simulink model "MJAUV_Maneuverability_model_V2"  (R2022b)
settings: Solver=ode4  StartTime=0.0  StopTime=50  FixedStep=0.0001  RelTol=1e-3  EnableMultiTasking=on
libraries: sharedutil x64, matrix_library x35
(part 1 of 5)
settings Model: Creator=Waqas Ali Waqar  LastModifiedBy=Administrator
settings SolverCC: ConcurrentTasks=on  ZeroCrossAlgorithm=Adaptive  AutoInsertRateTranBlk=on  InsertRTBMode=Never (minimum delay)
settings DataIOCC: SaveFormat=StructureWithTime
settings OptimizationCC: BlockReduction=off  OptimizeBlockIOStorage=off  BufferReuse=off  GlobalBufferReuse=off  ExpressionFolding=off  PassReuseOutputArgsThreshold=0  LocalBlockOutputs=off  OptimizeBlockOrder=speed  OptimizeDataStoreBuffers=off  BusAssignmentInplaceUpdate=off
settings DebuggingCC: IgnoredZcDiagnostic=none  ParameterTunabilityLossMsg=error  UnconnectedInputMsg=warning  UnconnectedOutputMsg=warning  UnconnectedLineMsg=warning
settings HardwareCC: ProdBitPerPointer=32  ProdBitPerSizeT=32  ProdBitPerPtrDiffT=32  ProdLargestAtomicFloat=None  ProdWordSize=32  ProdLongLongMode=on  ProdHWDeviceType=Generic->32-bit x86 compatible
settings ModelReferenceCC: EnableRefExpFcnMdlSchedulingChecks=on
settings SFSimCC: MATLABDynamicMemAlloc=off  CustomCodeUndefinedFunction=UseInterfaceOnly
settings RTWCC: GenerateReport=on  RTWVerbose=off  LaunchReport=on  RTWCompilerOptimization=on  DLArmComputeVersion=19.05
settings CodeAppCC: ForceParamTrailComments=on  OperatorAnnotations=on
settings GRTTargetCC: TargetLangStandard=C89/C90 (ANSI)

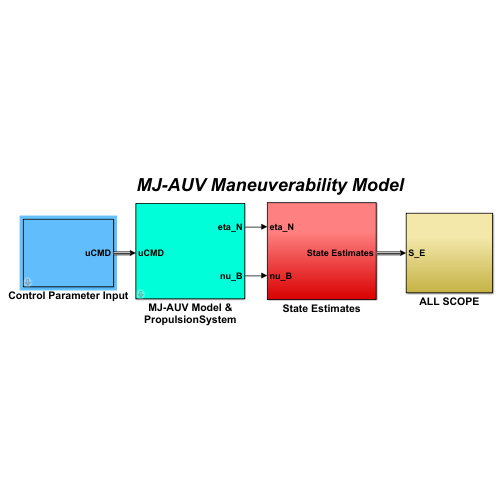
[thumbnail: Simulink's stored preview of the top-level diagram]
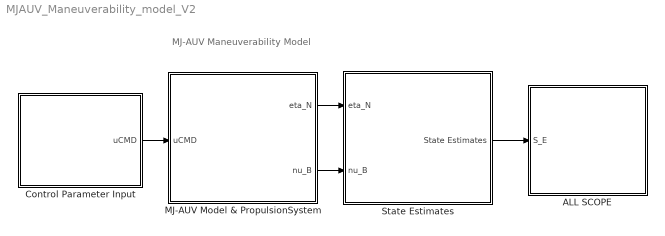
== system MJAUV_Maneuverability_model_V2 ==
  note: MJ-AUV Maneuverability Model
  ALL SCOPE : Subsystem
  Control Parameter Input : Subsystem  mask{uHT=50, uVT1=0, uVT2=0, Theta1=pi/60, Theta2=pi/60, Theta3=pi/60, x_rG_S=0, y_rG_S=0, z_rG_S=0, Delta_B_T=-2}
      mask prompts: uHT "uHT (rps)"; uVT1 "uVT1 (rad)"; uVT2 "uVT2 (rad)"; Theta1 "Theta1 (rad)"; Theta2 "Theta2 (rad)"; Theta3 "Theta3 (rad)"; Delta_B_T "Delta_B_T (N)"
      mask DialogControl ParameterGroupVar Prompt: Control Parameter Input
      mask DialogControl Container3 Prompt: rG_S
  MJ-AUV Model & PropulsionSystem : Subsystem  mask{R=0.15, rho=1025, g=9.8, cdf=0.5, cdt=1, DL=diag([0;0;0;0;0;0]), e1=[1;0;0], e2=[0;1;0], e3=[0;0;1], mB=38.58, IB=[0.434 0 0;0 1.126 0;0 0 1.126], LB=0.532, rG_B=[0;0;0], rB_B=[0;0;-0.01], l_B=[-0.532;0;0], r_B=[-0.532/2;0;0], B_B=377.7, W_B=377.7, mS=50.862, IS=[0.572 0 0;0 2.375 0;0 0 2.375], LS=0.702, rB_S=[0;0;-0.01], l_S=[-0.702;0;0], r_S=[-0.702/2;0;0], B_S=498.45, W_S=498.45, mT=50.862, IT=[0.572 0 0;0 2.375 0;0 0 2.375], LT=0.702, rG_T=[0;0;0], rB_T=[0;0;-0.01], l_T=[-0.702;0;0], r_T=[-0.702/2;0;0], W_T=498.45, mF=23.185, IF=[0.261 0 0;0 1.067 0;0 0 1.067], LF=0.320, rG_F=[0;0;0], rB_F=[0;0;-0.01], l_F=[-0.320;0;0], r_F=[-0.320/2;0;0], B_F=227.213, W_F=227.213, cL=0.5, xfin=-0.03, yfin=0.325, zfin=-0.045, alpha=0, Sfin=0.0421, r1=[-0.16;0;0], D=0.0762}
      mask prompts: R "Body Radius R"; rho "Seawater Density rho"; g "Acceleration of Gravity g"; cdf "Axial Drag Coefficient cdf"; cdt "Radial Drag Coefficient  cdt [0.8-1.2]"; DL "Linear Damping Matrix"; mB "Mass mB"; IB "Inertia Tensor IB"; LB "Length LB"; B_B "Buoyancy"; W_B "Weight"; mS "Mass mS"; IS "Inertia Tensor IS"; LS "Length LS"; rB_S "rB_B"; B_S "Buoyancy"; W_S "Weight"; mT "Mass mT"; IT "Inertia Tensor IT"; LT "Length LT"; W_T "Weight"; mF "Mass mF"; IF "Inertia Tensor IF"; LF "Length LF"; B_F "Buoyancy"; W_F "Weight"; cL "fin lift coefficient  cL:"; xfin "fin axial position xfin:"; yfin "fin axial position yfin:"; zfin "fin axial position zfin:"; alpha "fin flutter angle alpha"; Sfin "fin platform area Sfin:"; D "Diameter"
      mask init:
      | %%%%%%%%%%%%%%%%%%%%%%%%%%%%%%%%%%%%%%%%%%%%%%%%%%%%%%%
      | %%%%%%%%%%%%%%%%%%%  动力学  %%%%%%%%%%%%%%%%%%%%%%%%
      | %%%%%%%%%%%%%%%%%%%%%%%%%%%%%%%%%%%%%%%%%%%%%%%%%%%%%%%
      | 
      | 
      | %% JOINT-1
      | % 粘性水动力系数
      | Af = pi*R^2;
      | At_B = 2*pi*R*LB;
      | 
      | X_uu_B = rho*Af*cdf/2;
      | Y_vv_B = rho*At_B*cdt/2;
      | Z_ww_B = rho*At_B*cdt/2;
      | K_pp_B = 0;
      | M_qq_B = (rho*At_B*cdt*LB^3)/16;
      | N_rr_B = (rho*At_B*cdt*LB^3)/16;
      | 
      | dQ_B = -([X_uu_B;Y_vv_B;Z_ww_B;K_pp_B;M_qq_B;N_rr_B]);
      | 
      | 
      | %% JOINT-2
      | % 粘性水动力系数
      | Af = pi*R^2;
      | At_S = 2*pi*R*LS;
      | 
      | X_uu_S = rho*Af*cdf/2;
      | Y_vv_S = rho*At_S*cdt/2;
      | Z_ww_S = rho*At_S*cdt/2;
      | K_pp_S = 0;
      | M_qq_S = (rho*At_S*cdt*LS^3)/16;
      | N_rr_S = (rho*At_S*cdt*LS^3)/16;
      | 
      | dQ_S = -([X_uu_S;Y_vv_S;Z_ww_S;K_pp_S;M_qq_S;N_rr_S]);
      | 
      | %% JOINT-3
      | % 粘性水动力系数
      | Af = pi*R^2;
      | At_T = 2*pi*R*LT;
      | 
      | X_uu_T = rho*Af*cdf/2;
      | Y_vv_T = rho*At_T*cdt/2;
      | Z_ww_T = rho*At_T*cdt/2;
      | K_pp_T = 0;
      | M_qq_T = (rho*At_T*cdt*LT^3)/16;
      | N_rr_T = (rho*At_T*cdt*LT^3)/16;
      | 
      | dQ_T = -([X_uu_T;Y_vv_T;Z_ww_T;K_pp_T;M_qq_T;N_rr_T]);
      | 
      | 
      | %% JOINT-4
      | % 粘性水动力系数
      | Af = pi*R^2;
      | At_F = 2*pi*R*LF;
      | 
      | X_uu_F = rho*Af*cdf/2;
      | Y_vv_F = rho*At_F*cdt/2;
      | Z_ww_F = rho*At_F*cdt/2;
      | K_pp_F = 0;
      | M_qq_F = (rho*At_F*cdt*LF^3)/16;
      | N_rr_F = (rho*At_F*cdt*LF^3)/16;
      | 
      | dQ_F = -([X_uu_F;Y_vv_F;Z_ww_F;K_pp_F;M_qq_F;N_rr_F]);
      | 
      | 
      | 
      | %% 推进器
      | 
      | K = rho*D*D*D;
      | K_prop = [e1 ;skewsymm(r1)*e1]*K;
      mask DialogControl DescGroupVar Prompt: Paramteres and Variables
      mask DialogControl Container14 Prompt: Basic Parameters
      mask DialogControl Container17 Prompt: Joint-1 Parameters
      mask DialogControl Container17_copy Prompt: Joint-2 Parameters
      mask DialogControl Container17_copy_copy Prompt: Joint-3 Parameters
      mask DialogControl Container17_copy_copy_copy Prompt: Joint-4 Parameters
      mask DialogControl Container18 Prompt: Pectoral Fins Parameters
      mask DialogControl Container19 Prompt: Thrusters Parameters
  State Estimates : Subsystem
  wires:
  MJ-AUV Model & PropulsionSystem/2(nu_B) -> State Estimates/2(nu_B)
  MJ-AUV Model & PropulsionSystem/1(eta_N) -> State Estimates/1(eta_N)
  State Estimates/1(State Estimates) -> ALL SCOPE/1(S_E)
  Control Parameter Input/1(uCMD) -> MJ-AUV Model & PropulsionSystem/1(uCMD)

== system MJAUV_Maneuverability_model_V2/ALL SCOPE ==
  In Bus Element12 : Inport  PortName=S_E
  In Bus Element21 : Inport  PortName=S_E  Element=Position.Y
  In Bus Element22 : Inport  PortName=S_E  Element=Position.Z
  In Bus Element30 : Inport  PortName=S_E  Element=Position.Roll
  In Bus Element31 : Inport  PortName=S_E  Element=Position.Pitch
  In Bus Element32 : Inport  PortName=S_E  Element=Position.Yaw
  In Bus Element20 : Inport  PortName=S_E  Element=Position.X
  In Bus Element33 : Inport  PortName=S_E  Element=Velocity.u
  In Bus Element34 : Inport  PortName=S_E  Element=Velocity.v
  In Bus Element35 : Inport  PortName=S_E  Element=Velocity.w
  In Bus Element36 : Inport  PortName=S_E  Element=Velocity.p
  In Bus Element37 : Inport  PortName=S_E  Element=Velocity.q
  In Bus Element38 : Inport  PortName=S_E  Element=Velocity.r
  Roll/Pitch/Yaw (deg) : Scope  NumInputPorts=3
  To Workspace : Subsystem
  X/Y/Z (m) : Scope  NumInputPorts=3
  p/q/r (rad/s) : Scope  NumInputPorts=3
  u/v/w (m/s) : Scope  NumInputPorts=3
  wires:
  In Bus Element20/1 -> X/Y/Z (m)/1  "X"
  In Bus Element21/1 -> X/Y/Z (m)/2  "Y"
  In Bus Element22/1 -> X/Y/Z (m)/3  "Z"
  In Bus Element30/1 -> Roll/Pitch/Yaw (deg)/1  "Roll"
  In Bus Element31/1 -> Roll/Pitch/Yaw (deg)/2  "Pitch"
  In Bus Element32/1 -> Roll/Pitch/Yaw (deg)/3  "Yaw"
  In Bus Element33/1 -> u/v/w (m/s)/1  "u"
  In Bus Element34/1 -> u/v/w (m/s)/2  "v"
  In Bus Element35/1 -> u/v/w (m/s)/3  "w"
  In Bus Element36/1 -> p/q/r (rad/s)/1  "p"
  In Bus Element37/1 -> p/q/r (rad/s)/2  "q"
  In Bus Element38/1 -> p/q/r (rad/s)/3  "r"
  In Bus Element12/1 -> To Workspace/1(S_E)

== system MJAUV_Maneuverability_model_V2/Control Parameter Input ==
  Bus Creator2 : BusCreator  Inputs=4
  Constant7 : Constant  Value=Delta_B_T
  Saturation limits : Subsystem
  Subsystem : Subsystem
  Subsystem1 : Subsystem
  Subsystem2 : Subsystem
  uCMD : Outport
  wires:
  Bus Creator2/1 -> Saturation limits/1(InBus)
  Constant7/1 -> Bus Creator2/4  "Delta_B_T"
  Subsystem/1(uHT&VT) -> Bus Creator2/1
  Subsystem1/1(Theta) -> Bus Creator2/2
  Subsystem2/1(rG_S) -> Bus Creator2/3
  Saturation limits/1(uCMD) -> uCMD/1  "uHT uVT Theta rG_S Delta_B_T"

== system MJAUV_Maneuverability_model_V2/MJ-AUV Model & PropulsionSystem ==
  In Bus Element : Inport  PortName=uCMD
  Dynamics and Kinematics : Subsystem
      mask Display: image('$imagefile'); % 使用工具条上的 "编辑图像" 进行更改。
  Memory : Memory
  Propulsion System : Subsystem
  eta_N : Outport  VectorParamsAs1DForOutWhenUnconnected=off
  nu_B : Outport  Port=2  VectorParamsAs1DForOutWhenUnconnected=off
  wires:
  Dynamics and Kinematics/1(nu_B) -> Memory/1, nu_B/1  "[u    v    w    p    q    r]"
  Dynamics and Kinematics/2(eta_N) -> eta_N/1  "[x   y   z  q0  q1  q2  q3]"
  Propulsion System/1(Tau_HT) -> Dynamics and Kinematics/1(Tau_HT)
  Memory/1 -> Propulsion System/1(nu_B)
  Propulsion System/2(Tau_VT1&VT2) -> Dynamics and Kinematics/2(Tau_VT1&VT2)
  In Bus Element/1 -> Dynamics and Kinematics/3(uCMD), Propulsion System/2(uCMD)

== system MJAUV_Maneuverability_model_V2/State Estimates ==
  eta_N : Inport
  nu_B : Inport  Port=2
  Gain : Gain  Gain=180/pi
  Mux : Mux  Inputs=2
  Quaternions to Euler Angles : Subsystem
  eta1_E=[x,y,z] : Selector  InputPortWidth=7  IndexOptions=Index vector (dialog)  Indices=[1 2 3]  OutputSizes=1
  eta2_E=[q0,q1,q2,q3] : Selector  InputPortWidth=7  IndexOptions=Index vector (dialog)  Indices=[4 5 6 7]  OutputSizes=1
  signal transformation : Subsystem
  State Estimates : Outport  VectorParamsAs1DForOutWhenUnconnected=off
  wires:
  Gain/1 -> Mux/2
  signal transformation/1(State Estimate) -> State Estimates/1
  eta1_E=[x,y,z]/1 -> Mux/1
  Quaternions to Euler Angles/1(Euler Angles) -> Gain/1
  Mux/1 -> signal transformation/1(Position)
  eta2_E=[q0,q1,q2,q3]/1 -> Quaternions to Euler Angles/1(Quaternions)
  nu_B/1 -> signal transformation/2(nu_B)
  eta_N/1 -> eta1_E=[x,y,z]/1, eta2_E=[q0,q1,q2,q3]/1  "[x   y   z  q0  q1  q2  q3]"

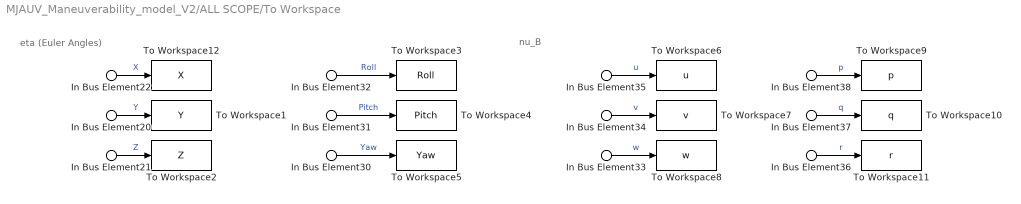
== system MJAUV_Maneuverability_model_V2/ALL SCOPE/To Workspace ==
  note: nu_B
  note: eta (Euler Angles)
  In Bus Element20 : Inport  PortName=S_E  Element=Position.Y
  In Bus Element21 : Inport  PortName=S_E  Element=Position.Z
  In Bus Element32 : Inport  PortName=S_E  Element=Position.Roll
  In Bus Element31 : Inport  PortName=S_E  Element=Position.Pitch
  In Bus Element30 : Inport  PortName=S_E  Element=Position.Yaw
  In Bus Element22 : Inport  PortName=S_E  Element=Position.X
  In Bus Element35 : Inport  PortName=S_E  Element=Velocity.u
  In Bus Element34 : Inport  PortName=S_E  Element=Velocity.v
  In Bus Element33 : Inport  PortName=S_E  Element=Velocity.w
  In Bus Element38 : Inport  PortName=S_E  Element=Velocity.p
  In Bus Element37 : Inport  PortName=S_E  Element=Velocity.q
  In Bus Element36 : Inport  PortName=S_E  Element=Velocity.r
  To Workspace1 : ToWorkspace  VariableName=Y  SampleTime=-1
  To Workspace10 : ToWorkspace  VariableName=q  SampleTime=-1
  To Workspace11 : ToWorkspace  VariableName=r  SampleTime=-1
  To Workspace12 : ToWorkspace  VariableName=X  SampleTime=-1
  To Workspace2 : ToWorkspace  VariableName=Z  SampleTime=-1
  To Workspace3 : ToWorkspace  VariableName=Roll  SampleTime=-1
  To Workspace4 : ToWorkspace  VariableName=Pitch  SampleTime=-1
  To Workspace5 : ToWorkspace  VariableName=Yaw  SampleTime=-1
  To Workspace6 : ToWorkspace  VariableName=u  SampleTime=-1
  To Workspace7 : ToWorkspace  VariableName=v  SampleTime=-1
  To Workspace8 : ToWorkspace  VariableName=w  SampleTime=-1
  To Workspace9 : ToWorkspace  VariableName=p  SampleTime=-1
  wires:
  In Bus Element21/1 -> To Workspace2/1  "Z"
  In Bus Element22/1 -> To Workspace12/1  "X"
  In Bus Element35/1 -> To Workspace6/1  "u"
  In Bus Element33/1 -> To Workspace8/1  "w"
  In Bus Element38/1 -> To Workspace9/1  "p"
  In Bus Element31/1 -> To Workspace4/1  "Pitch"
  In Bus Element37/1 -> To Workspace10/1  "q"
  In Bus Element36/1 -> To Workspace11/1  "r"
  In Bus Element32/1 -> To Workspace3/1  "Roll"
  In Bus Element30/1 -> To Workspace5/1  "Yaw"
  In Bus Element34/1 -> To Workspace7/1  "v"
  In Bus Element20/1 -> To Workspace1/1  "Y"

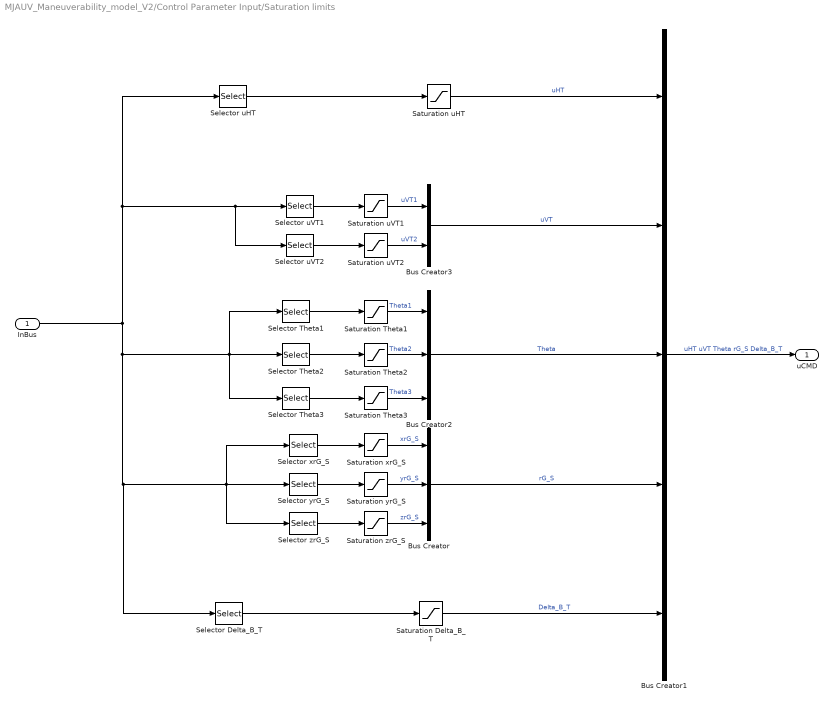
== system MJAUV_Maneuverability_model_V2/Control Parameter Input/Saturation limits ==
  InBus : Inport
  Bus Creator : BusCreator  Inputs=3
  Bus Creator1 : BusCreator  Inputs=5
  Bus Creator2 : BusCreator  Inputs=3
  Bus Creator3 : BusCreator  Inputs=2
  Saturation Delta_B_T : Saturate  UpperLimit=10  LowerLimit=-10
  Saturation Theta1 : Saturate  UpperLimit=pi/6  LowerLimit=-pi/6
  Saturation Theta2 : Saturate  UpperLimit=pi/6  LowerLimit=-pi/6
  Saturation Theta3 : Saturate  UpperLimit=pi/6  LowerLimit=-pi/6
  Saturation uHT : Saturate  UpperLimit=60  LowerLimit=0
  Saturation uVT1 : Saturate  UpperLimit=pi/3  LowerLimit=-pi/3
  Saturation uVT2 : Saturate  UpperLimit=pi/3  LowerLimit=-pi/3
  Saturation xrG_S : Saturate  UpperLimit=0.1  LowerLimit=-0.1
  Saturation yrG_S : Saturate  UpperLimit=0.1  LowerLimit=-0.1
  Saturation zrG_S : Saturate  UpperLimit=0.1  LowerLimit=-0.1
  Selector Delta_B_T : Selector  InputPortWidth=10  IndexOptions=Index vector (dialog)  Indices=[10]  OutputSizes=1
  Selector Theta1 : Selector  InputPortWidth=10  IndexOptions=Index vector (dialog)  Indices=[4]  OutputSizes=1
  Selector Theta2 : Selector  InputPortWidth=10  IndexOptions=Index vector (dialog)  Indices=[5]  OutputSizes=1
  Selector Theta3 : Selector  InputPortWidth=10  IndexOptions=Index vector (dialog)  Indices=[6]  OutputSizes=1
  Selector uHT : Selector  InputPortWidth=10  IndexOptions=Index vector (dialog)  Indices=[1]  OutputSizes=1
  Selector uVT1 : Selector  InputPortWidth=10  IndexOptions=Index vector (dialog)  Indices=[2]  OutputSizes=1
  Selector uVT2 : Selector  InputPortWidth=10  IndexOptions=Index vector (dialog)  Indices=[3]  OutputSizes=1
  Selector xrG_S : Selector  InputPortWidth=10  IndexOptions=Index vector (dialog)  Indices=[7]  OutputSizes=1
  Selector yrG_S : Selector  InputPortWidth=10  IndexOptions=Index vector (dialog)  Indices=[8]  OutputSizes=1
  Selector zrG_S : Selector  InputPortWidth=10  IndexOptions=Index vector (dialog)  Indices=[9]  OutputSizes=1
  uCMD : Outport  VectorParamsAs1DForOutWhenUnconnected=off
  wires:
  Bus Creator1/1 -> uCMD/1  "uHT uVT Theta rG_S Delta_B_T"
  Selector zrG_S/1 -> Saturation zrG_S/1
  Selector yrG_S/1 -> Saturation yrG_S/1
  Selector xrG_S/1 -> Saturation xrG_S/1
  Saturation xrG_S/1 -> Bus Creator/1  "xrG_S"
  Saturation yrG_S/1 -> Bus Creator/2  "yrG_S"
  Saturation zrG_S/1 -> Bus Creator/3  "zrG_S"
  Bus Creator/1 -> Bus Creator1/4  "rG_S"
  Selector Theta2/1 -> Saturation Theta2/1
  Selector Theta1/1 -> Saturation Theta1/1
  Selector Theta3/1 -> Saturation Theta3/1
  Saturation Theta1/1 -> Bus Creator2/1  "Theta1"
  Saturation Theta2/1 -> Bus Creator2/2  "Theta2"
  Saturation Theta3/1 -> Bus Creator2/3  "Theta3"
  Bus Creator2/1 -> Bus Creator1/3  "Theta"
  Saturation uVT1/1 -> Bus Creator3/1  "uVT1"
  Saturation uVT2/1 -> Bus Creator3/2  "uVT2"
  Selector uVT2/1 -> Saturation uVT2/1
  Selector uVT1/1 -> Saturation uVT1/1
  Bus Creator3/1 -> Bus Creator1/2  "uVT"
  Selector uHT/1 -> Saturation uHT/1
  Saturation uHT/1 -> Bus Creator1/1  "uHT"
  Selector Delta_B_T/1 -> Saturation Delta_B_T/1
  InBus/1 -> Selector uVT2/1, Selector uVT1/1, Selector uHT/1, Selector Theta3/1, Selector Theta1/1, Selector Theta2/1, Selector zrG_S/1, Selector xrG_S/1, Selector yrG_S/1, Selector Delta_B_T/1
  Saturation Delta_B_T/1 -> Bus Creator1/5  "Delta_B_T"

== system MJAUV_Maneuverability_model_V2/Control Parameter Input/Subsystem ==
  Bus Creator : BusCreator  Inputs=3
  Constant1 : Constant  Value=uHT
  Constant2 : Constant  Value=uVT1
  Constant3 : Constant  Value=uVT2
  uHT&VT : Outport
  wires:
  Constant2/1 -> Bus Creator/2  "uVT1"
  Constant3/1 -> Bus Creator/3  "uVT2"
  Constant1/1 -> Bus Creator/1  "uHT"
  Bus Creator/1 -> uHT&VT/1  "uHT&VT"

== system MJAUV_Maneuverability_model_V2/Control Parameter Input/Subsystem1 ==
  Bus Creator1 : BusCreator  Inputs=3
  Constant : Constant  Value=Theta2
  Constant4 : Constant  Value=Theta1
  Constant5 : Constant  Value=Theta3
  Theta : Outport
  wires:
  Constant4/1 -> Bus Creator1/1  "Theta1"
  Constant/1 -> Bus Creator1/2  "Theta2"
  Constant5/1 -> Bus Creator1/3  "Theta3"
  Bus Creator1/1 -> Theta/1  "Theta"

== system MJAUV_Maneuverability_model_V2/Control Parameter Input/Subsystem2 ==
  Bus Creator : BusCreator  Inputs=3
  Constant1 : Constant  Value=y_rG_S
  Constant2 : Constant  Value=z_rG_S
  Constant6 : Constant  Value=x_rG_S
  rG_S : Outport
  wires:
  Constant1/1 -> Bus Creator/2  "y_rG_S"
  Constant6/1 -> Bus Creator/1  "x_rG_S"
  Constant2/1 -> Bus Creator/3  "z_rG_S"
  Bus Creator/1 -> rG_S/1  "rG_S"

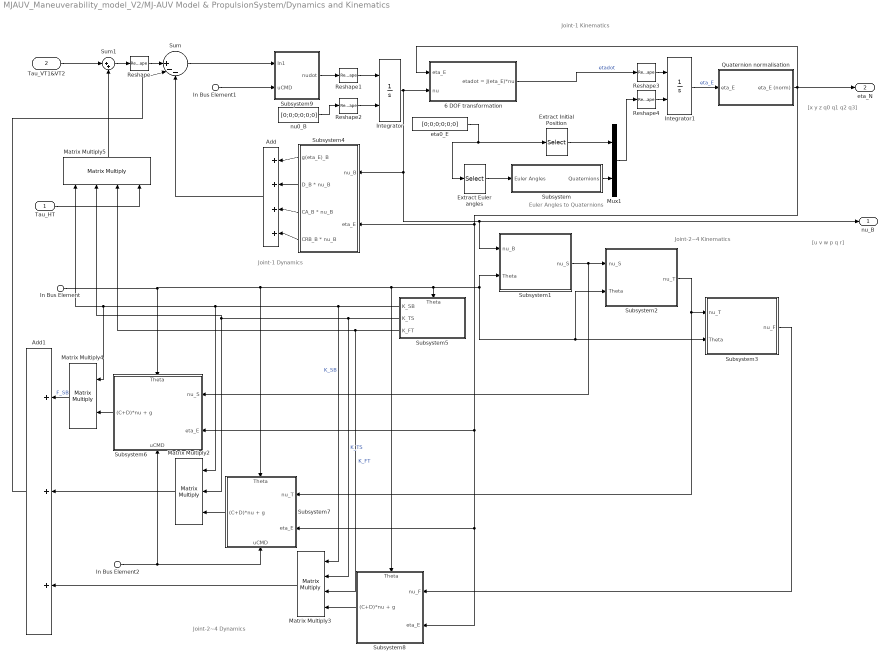
== system MJAUV_Maneuverability_model_V2/MJ-AUV Model & PropulsionSystem/Dynamics and Kinematics ==
  note: Joint-1 Dynamics
  note: [u v w p q r]
  note: [x y z q0 q1 q2 q3]
  note: Euler Angles to Quaternions
  note: Joint-1 Kinematics
  note: Joint-2~4 Kinematics
  note: Joint-2~4 Dynamics
  Tau_HT : Inport
  Tau_VT1&VT2 : Inport  Port=2
  In Bus Element1 : Inport  Port=3  PortName=uCMD
  In Bus Element2 : Inport  Port=3  PortName=uCMD
  In Bus Element : Inport  Port=3  PortName=uCMD  Element=Theta
  6 DOF transformation : Subsystem
  Add : Sum  Inputs=++++
  Add1 : Sum  Inputs=+++
  Extract Euler angles : Selector  InputPortWidth=6  IndexOptions=Index vector (dialog)  Indices=[4 5 6]  OutputSizes=1
  Extract Initial Position : Selector  InputPortWidth=6  IndexOptions=Index vector (dialog)  Indices=[1 2 3]  OutputSizes=1
  Integrator : Integrator  InitialConditionSource=external
  Integrator1 : Integrator  InitialConditionSource=external
  Matrix Multiply2 : Product  Inputs=3  Multiplication=Matrix(*)
  Matrix Multiply3 : Product  Inputs=4  Multiplication=Matrix(*)
  Matrix Multiply4 : Product  Multiplication=Matrix(*)
  Matrix Multiply5 : Product  Inputs=4  Multiplication=Matrix(*)
  Mux1 : Mux  Inputs=2
  Quaternion normalisation : Subsystem
  Reshape{,1..4} (5 alike) : Reshape  OutputDimensionality=Column vector (2-D)
  Subsystem : Subsystem
  Subsystem1 : Subsystem
  Subsystem2 : Subsystem
  Subsystem3 : Subsystem
  Subsystem4 : Subsystem
  Subsystem5 : Subsystem
      settings: PortSchema="{\"entries\":[{\"content\":{\"sides\":[{\"content\":{\"connectorIds\":[]},\"type\":\"ConnectorPlacement.EquallySpacedRectSide\",\"uuid\":\"71b21129-4088-44fc-819a-967612d65132\"},{\"content\":{\"connectorIds\":[\"Out1\",\"Out2\",\"Out3\"],\"side\":\"RIGHT\"},\"type\":\"ConnectorPlacement.EquallySpacedRectSide\",\"uuid\":\"a2be8efb-ce7d-47fd-a29f-307f4b0a3364\"},{\"content\":{\"connectorIds\":[\"In1\"],\"side\":\"TOP\"},\"type\":\"ConnectorPlacement.EquallySpacedRectSide\",\"uuid\":\"eaff307d-2c91-4f60-8388-37c57609f459\"}]},\"type\":\"ConnectorPlacement.EquallySpacedConnector\",\"uuid\":\"fafd8f31-37dd-46d8-bc19-86e5d3c9fd42\"}],\"packageUris\":[\"http://schema.mathworks.com/mf0/Connector/R2020b\"],\"version\":\"1.0\"}"
  Subsystem6 : Subsystem
      settings: PortSchema="{\"entries\":[{\"content\":{\"sides\":[{\"content\":{\"connectorIds\":[\"In1\",\"In2\"]},\"type\":\"ConnectorPlacement.EquallySpacedRectSide\",\"uuid\":\"2992bc57-63bf-42d7-8a1f-c728ab5ac8fb\"},{\"content\":{\"connectorIds\":[\"Out1\"],\"side\":\"RIGHT\"},\"type\":\"ConnectorPlacement.EquallySpacedRectSide\",\"uuid\":\"6befd73f-bf7d-4fcc-a749-cb84c3a0eaa3\"},{\"content\":{\"connectorIds\":[\"In3\"],\"side\":\"TOP\"},\"type\":\"ConnectorPlacement.EquallySpacedRectSide\",\"uuid\":\"3258d01b-5179-4970-b54d-ce72a38fec34\"},{\"content\":{\"connectorIds\":[\"In4\"],\"side\":\"BOTTOM\"},\"type\":\"ConnectorPlacement.EquallySpacedRectSide\",\"uuid\":\"c2ea7583-5795-47d0-9926-ba142740563b\"}]},\"type\":\"ConnectorPlacement.EquallySpacedConnector\",\"uuid\":\"e1edb069-49c6-4d27-bce8-a67f8d43e2ed\"}],\"packageUris\":[\"http://schema.mathworks.com/mf0/Connector/R2020b\"],\"version\":\"1.0\"}"
  Subsystem7 : Subsystem
      settings: PortSchema="{\"entries\":[{\"content\":{\"sides\":[{\"content\":{\"connectorIds\":[\"In1\",\"In2\"]},\"type\":\"ConnectorPlacement.EquallySpacedRectSide\",\"uuid\":\"31af84fe-62b1-4301-ba62-b0ce42dbbe74\"},{\"content\":{\"connectorIds\":[\"Out1\"],\"side\":\"RIGHT\"},\"type\":\"ConnectorPlacement.EquallySpacedRectSide\",\"uuid\":\"9c52d008-6ea2-410e-9598-64e81901bbd4\"},{\"content\":{\"connectorIds\":[\"In3\"],\"side\":\"TOP\"},\"type\":\"ConnectorPlacement.EquallySpacedRectSide\",\"uuid\":\"52b5cbd7-9b57-449e-a08a-13cbcc88606c\"},{\"content\":{\"connectorIds\":[\"In4\"],\"side\":\"BOTTOM\"},\"type\":\"ConnectorPlacement.EquallySpacedRectSide\",\"uuid\":\"92c6015e-158f-400b-84e6-8a887d96aa28\"}]},\"type\":\"ConnectorPlacement.EquallySpacedConnector\",\"uuid\":\"e37ef176-498d-4e2c-a052-68648f7e7e95\"}],\"packageUris\":[\"http://schema.mathworks.com/mf0/Connector/R2020b\"],\"version\":\"1.0\"}"
  Subsystem8 : Subsystem
      settings: PortSchema="{\"entries\":[{\"content\":{\"sides\":[{\"content\":{\"connectorIds\":[\"In1\",\"In2\"]},\"type\":\"ConnectorPlacement.EquallySpacedRectSide\",\"uuid\":\"31af84fe-62b1-4301-ba62-b0ce42dbbe74\"},{\"content\":{\"connectorIds\":[\"Out1\"],\"side\":\"RIGHT\"},\"type\":\"ConnectorPlacement.EquallySpacedRectSide\",\"uuid\":\"9c52d008-6ea2-410e-9598-64e81901bbd4\"},{\"content\":{\"connectorIds\":[\"In3\"],\"side\":\"TOP\"},\"type\":\"ConnectorPlacement.EquallySpacedRectSide\",\"uuid\":\"52b5cbd7-9b57-449e-a08a-13cbcc88606c\"}]},\"type\":\"ConnectorPlacement.EquallySpacedConnector\",\"uuid\":\"e37ef176-498d-4e2c-a052-68648f7e7e95\"}],\"packageUris\":[\"http://schema.mathworks.com/mf0/Connector/R2020b\"],\"version\":\"1.0\"}"
  Subsystem9 : Subsystem
  Sum : Sum  Inputs=||+--  SaturateOnIntegerOverflow=on
  Sum1 : Sum  Inputs=|++
  eta0_E : Constant  Value=[0;0;0;0;0;0]
  nu0_B : Constant  Value=[0;0;0;0;0;0]
  nu_B : Outport  VectorParamsAs1DForOutWhenUnconnected=off
  eta_N : Outport  Port=2  VectorParamsAs1DForOutWhenUnconnected=off
  wires:
  Reshape3/1 -> Integrator1/1
  Reshape2/1 -> Integrator/2
  nu0_B/1 -> Reshape2/1
  6 DOF transformation/1(etadot = J(eta_E)*nu) -> Reshape3/1  "etadot"
  Integrator1/1 -> Quaternion normalisation/1(eta_E)  "eta_E"
  Reshape/1 -> Sum/1
  Extract Euler angles/1 -> Subsystem/1("Euler Angles ")
  Mux1/1 -> Reshape4/1
  Reshape4/1 -> Integrator1/2
  Extract Initial Position/1 -> Mux1/1
  eta0_E/1 -> Extract Initial Position/1, Extract Euler angles/1
  Subsystem/1(Quaternions) -> Mux1/2
  In Bus Element/1 -> Subsystem3/2(Theta), Subsystem2/2(Theta), Subsystem1/2(Theta), Subsystem5/1(Theta), Subsystem8/3(Theta), Subsystem7/3(Theta), Subsystem6/3(Theta)
  Subsystem4/1(g(eta_E)_B) -> Add/1
  Subsystem4/2(D_B * nu_B) -> Add/2
  Subsystem4/3(CA_B * nu_B) -> Add/3
  Subsystem4/4(CRB_B * nu_B) -> Add/4
  Subsystem8/1((C+D)*nu + g) -> Matrix Multiply3/4
  Subsystem5/3(K_FT) -> Matrix Multiply5/3, Matrix Multiply3/3  "K_FT"
  Subsystem2/1(nu_T) -> Subsystem3/1(nu_T), Subsystem7/1(nu_T)
  Subsystem3/1(nu_F) -> Subsystem8/1(nu_F)
  Subsystem1/1(nu_S) -> Subsystem2/1(nu_S), Subsystem6/1(nu_S)
  Matrix Multiply3/1 -> Add1/3
  Add/1 -> Sum/3
  Subsystem7/1((C+D)*nu + g) -> Matrix Multiply2/3
  Subsystem5/2(K_TS) -> Matrix Multiply5/2, Matrix Multiply2/2, Matrix Multiply3/2  "K_TS"
  Matrix Multiply2/1 -> Add1/2
  Subsystem5/1(K_SB) -> Matrix Multiply5/1, Matrix Multiply4/1, Matrix Multiply2/1, Matrix Multiply3/1  "K_SB"
  Subsystem6/1((C+D)*nu + g) -> Matrix Multiply4/2
  Integrator/1 -> Subsystem1/1(nu_B), nu_B/1, Subsystem4/1(nu_B), 6 DOF transformation/2(nu)
  Reshape1/1 -> Integrator/1
  Quaternion normalisation/1(eta_E (norm)) -> eta_N/1, 6 DOF transformation/1(eta_E), Subsystem8/2(eta_E), Subsystem7/2(eta_E), Subsystem6/2(eta_E), Subsystem4/2(eta_E)
  Add1/1 -> Sum/2
  Sum/1 -> Subsystem9/1(In1)
  Subsystem9/1(nudot) -> Reshape1/1
  Tau_HT/1 -> Matrix Multiply5/4
  Matrix Multiply5/1 -> Sum1/2
  Sum1/1 -> Reshape/1
  Tau_VT1&VT2/1 -> Sum1/1
  Matrix Multiply4/1 -> Add1/1  "F_SB"
  In Bus Element1/1 -> Subsystem9/2(uCMD)
  In Bus Element2/1 -> Subsystem6/4(uCMD), Subsystem7/4(uCMD)

== system MJAUV_Maneuverability_model_V2/MJ-AUV Model & PropulsionSystem/Propulsion System ==
  note: square
  nu_B : Inport
  In Bus Element2 : Inport  Port=2  PortName=uCMD  Element=uHT
  In Bus Element1 : Inport  Port=2  PortName=uCMD  Element=uVT
  Horizontal Force and Moment (Tau_H) : Subsystem
  Vertical Force and Moment (Tau_V) : Subsystem
  Tau_HT : Outport  VectorParamsAs1DForOutWhenUnconnected=off
  Tau_VT1&VT2 : Outport  Port=2  VectorParamsAs1DForOutWhenUnconnected=off
  wires:
  Vertical Force and Moment (Tau_V)/1("Tau_VT1&VT2 ") -> Tau_VT1&VT2/1
  Horizontal Force and Moment (Tau_H)/1(Tau_HT) -> Tau_HT/1
  nu_B/1 -> Vertical Force and Moment (Tau_V)/1(nu_B), Horizontal Force and Moment (Tau_H)/2(nu_B)
  In Bus Element2/1 -> Horizontal Force and Moment (Tau_H)/1(uHT)
  In Bus Element1/1 -> Vertical Force and Moment (Tau_V)/2(uVT)

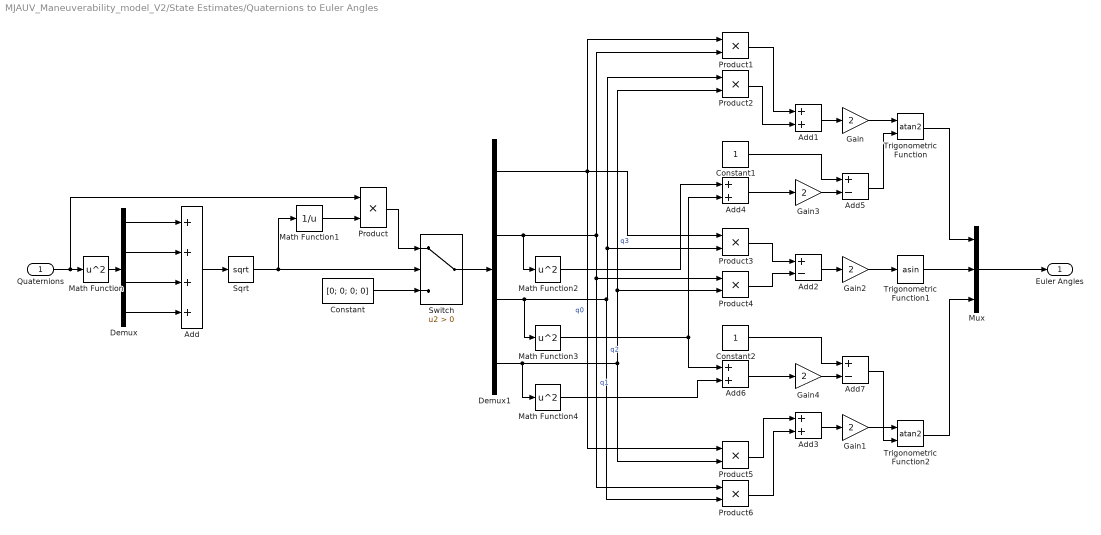
== system MJAUV_Maneuverability_model_V2/State Estimates/Quaternions to Euler Angles ==
  Quaternions : Inport
  Add : Sum  Inputs=4
  Add{1,3..4,6} (4 alike) : Sum
  Add2 : Sum  Inputs=+-
  Add5 : Sum  Inputs=+-
  Add7 : Sum  Inputs=+-
  Constant : Constant  Value=[0; 0; 0; 0]
  Constant1 : Constant
  Constant2 : Constant
  Demux : Demux
  Demux1 : Demux
  Gain{,1..4} (5 alike) : Gain  Gain=2
  Math Function{,2..4} (4 alike) : Math  Operator=square  SignedPower=on
  Math Function1 : Math  Operator=reciprocal  SignedPower=on
  Mux : Mux  Inputs=3
  Product{,1..6} (7 alike) : Product
  Sqrt : Sqrt
  Switch : Switch  Criteria=u2 > Threshold  SaturateOnIntegerOverflow=off  InputSameDT=off
  Trigonometric Function : Trigonometry  Operator=atan2
  Trigonometric Function1 : Trigonometry  Operator=asin
  Trigonometric Function2 : Trigonometry  Operator=atan2
  Euler Angles : Outport  VectorParamsAs1DForOutWhenUnconnected=off
  wires:
  Quaternions/1 -> Product/1, Math Function/1
  Add/1 -> Sqrt/1
  Sqrt/1 -> Math Function1/1, Switch/2
  Constant/1 -> Switch/3
  Math Function1/1 -> Product/2
  Product/1 -> Switch/1
  Switch/1 -> Demux1/1
  Demux1/1 -> Product5/1, Product3/1, Product1/1  "q0"
  Demux1/2 -> Product6/1, Product4/1, Product1/2, Math Function2/1  "q1"
  Demux1/3 -> Product6/2, Product3/2, Product2/1, Math Function3/1  "q2"
  Demux1/4 -> Product5/2, Product4/2, Product2/2, Math Function4/1  "q3"
  Trigonometric Function1/1 -> Mux/2
  Mux/1 -> Euler Angles/1
  Trigonometric Function/1 -> Mux/1
  Trigonometric Function2/1 -> Mux/3
  Gain/1 -> Trigonometric Function/1
  Gain1/1 -> Trigonometric Function2/1
  Gain2/1 -> Trigonometric Function1/1
  Add1/1 -> Gain/1
  Add2/1 -> Gain2/1
  Add3/1 -> Gain1/1
  Product3/1 -> Add2/1
  Product4/1 -> Add2/2
  Product5/1 -> Add3/1
  Product6/1 -> Add3/2
  Product2/1 -> Add1/2
  Product1/1 -> Add1/1
  Add4/1 -> Gain3/1
  Gain3/1 -> Add5/2
  Constant1/1 -> Add5/1
  Add5/1 -> Trigonometric Function/2
  Add7/1 -> Trigonometric Function2/2
  Add6/1 -> Gain4/1
  Gain4/1 -> Add7/2
  Constant2/1 -> Add7/1
  Math Function2/1 -> Add4/1
  Math Function3/1 -> Add6/1, Add4/2
  Math Function4/1 -> Add6/2
  Demux/1 -> Add/1
  Demux/2 -> Add/2
  Demux/3 -> Add/3
  Demux/4 -> Add/4
  Math Function/1 -> Demux/1

== system MJAUV_Maneuverability_model_V2/State Estimates/signal transformation ==
  Position : Inport
  nu_B : Inport  Port=2
  Bus Creator : BusCreator  Inputs=6
  Bus Creator1 : BusCreator  Inputs=6
  Bus Creator2 : BusCreator  Inputs=2
  Selector : Selector  InputPortWidth=6  IndexOptions=Index vector (dialog)  Indices=[1]  OutputSizes=1
  Selector1 : Selector  InputPortWidth=6  IndexOptions=Index vector (dialog)  Indices=[2]  OutputSizes=1
  Selector10 : Selector  InputPortWidth=6  IndexOptions=Index vector (dialog)  Indices=[5]  OutputSizes=1
  Selector11 : Selector  InputPortWidth=6  IndexOptions=Index vector (dialog)  Indices=[6]  OutputSizes=1
  Selector2 : Selector  InputPortWidth=6  IndexOptions=Index vector (dialog)  Indices=[3]  OutputSizes=1
  Selector3 : Selector  InputPortWidth=6  IndexOptions=Index vector (dialog)  Indices=[4]  OutputSizes=1
  Selector4 : Selector  InputPortWidth=6  IndexOptions=Index vector (dialog)  Indices=[5]  OutputSizes=1
  Selector5 : Selector  InputPortWidth=6  IndexOptions=Index vector (dialog)  Indices=[6]  OutputSizes=1
  Selector6 : Selector  InputPortWidth=6  IndexOptions=Index vector (dialog)  Indices=[1]  OutputSizes=1
  Selector7 : Selector  InputPortWidth=6  IndexOptions=Index vector (dialog)  Indices=[2]  OutputSizes=1
  Selector8 : Selector  InputPortWidth=6  IndexOptions=Index vector (dialog)  Indices=[3]  OutputSizes=1
  Selector9 : Selector  InputPortWidth=6  IndexOptions=Index vector (dialog)  Indices=[4]  OutputSizes=1
  State Estimate : Outport  VectorParamsAs1DForOutWhenUnconnected=off
  wires:
  Position/1 -> Selector5/1, Selector4/1, Selector3/1, Selector2/1, Selector1/1, Selector/1
  Selector/1 -> Bus Creator/1  "X"
  Selector1/1 -> Bus Creator/2  "Y"
  Selector2/1 -> Bus Creator/3  "Z"
  Selector3/1 -> Bus Creator/4  "Roll"
  Selector4/1 -> Bus Creator/5  "Pitch"
  nu_B/1 -> Selector8/1, Selector7/1, Selector6/1, Selector11/1, Selector10/1, Selector9/1
  Selector6/1 -> Bus Creator1/1  "u"
  Selector7/1 -> Bus Creator1/2  "v"
  Selector8/1 -> Bus Creator1/3  "w"
  Selector9/1 -> Bus Creator1/4  "p"
  Selector10/1 -> Bus Creator1/5  "q"
  Selector11/1 -> Bus Creator1/6  "r"
  Bus Creator/1 -> Bus Creator2/1  "Position"
  Bus Creator1/1 -> Bus Creator2/2  "Velocity"
  Bus Creator2/1 -> State Estimate/1
  Selector5/1 -> Bus Creator/6  "Yaw"

== system MJAUV_Maneuverability_model_V2/MJ-AUV Model & PropulsionSystem/Dynamics and Kinematics/6 DOF transformation ==
  note: eta2dot
  note: eta1dot
  note: e=[eta;e1;e2;e3]
  note: u v w
  note: p q r
  eta_E : Inport
  nu : Inport  Port=2
  E1(e) : Subsystem
  E2(e) : Subsystem
  Mux : Mux  Inputs=2
  Product : Product  Inputs=**  Multiplication=Matrix(*)  SaturateOnIntegerOverflow=on  OutDataTypeStr=Inherit: Same as first input
  Product1 : Product  Inputs=**  Multiplication=Matrix(*)  SaturateOnIntegerOverflow=on  OutDataTypeStr=Inherit: Same as first input
  Selector : Selector  InputPortWidth=7  IndexOptions=Index vector (dialog)  Indices=[4 5 6 7]  OutputSizes=1
  Selector1 : Selector  InputPortWidth=6  IndexOptions=Index vector (dialog)  Indices=[1 2 3]  OutputSizes=1
  Selector2 : Selector  InputPortWidth=6  IndexOptions=Index vector (dialog)  Indices=[4 5 6]  OutputSizes=1
  etadot = J(eta_E)*nu : Outport  VectorParamsAs1DForOutWhenUnconnected=off
  wires:
  Selector/1 -> E2(e)/1(e), E1(e)/1(e)
  eta_E/1 -> Selector/1
  E1(e)/1(E1) -> Product/1
  nu/1 -> Selector1/1, Selector2/1
  Selector1/1 -> Product/2
  Selector2/1 -> Product1/2
  E2(e)/1(E2) -> Product1/1
  Product/1 -> Mux/1
  Mux/1 -> etadot = J(eta_E)*nu/1
  Product1/1 -> Mux/2

== system MJAUV_Maneuverability_model_V2/MJ-AUV Model & PropulsionSystem/Dynamics and Kinematics/Quaternion normalisation ==
  eta_E : Inport
  Mux : Mux  Inputs=2
  Product : Product  Inputs=*/  SaturateOnIntegerOverflow=on  OutDataTypeStr=Inherit: Same as first input
  Reshape : Reshape  OutputDimensionality=Column vector (2-D)
  Selector : Selector  InputPortWidth=7  IndexOptions=Index vector (dialog)  Indices=[1 2 3]  OutputSizes=1
  Selector1 : Selector  InputPortWidth=7  IndexOptions=Index vector (dialog)  Indices=[4 5 6 7]  OutputSizes=1
  norm 1x4 vector : Subsystem
  eta_E (norm) : Outport  VectorParamsAs1DForOutWhenUnconnected=off
  wires:
  norm 1x4 vector/1(norm) -> Product/2
  Reshape/1 -> eta_E (norm)/1
  Mux/1 -> Reshape/1
  Product/1 -> Mux/2
  Selector/1 -> Mux/1
  Selector1/1 -> Product/1, norm 1x4 vector/1(Inport)
  eta_E/1 -> Selector/1, Selector1/1  "eta_E"

== system MJAUV_Maneuverability_model_V2/MJ-AUV Model & PropulsionSystem/Dynamics and Kinematics/Subsystem ==
  "Euler Angles " : Inport
  Add : Sum
  Add1 : Sum  Inputs=-+
  Add2 : Sum
  Add3 : Sum  Inputs=+-
  Demux : Demux  Outputs=3
  Demux1 : Demux  Outputs=3
  Gain : Gain  Gain=0.5
  Mux : Mux
  Product{,1..7} (8 alike) : Product  Inputs=3
  Trigonometric Function : Trigonometry
  Trigonometric Function1 : Trigonometry  Operator=cos
  Quaternions : Outport  VectorParamsAs1DForOutWhenUnconnected=off
  wires:
  Add3/1 -> Mux/4
  Add2/1 -> Mux/3
  Add/1 -> Mux/1
  Add1/1 -> Mux/2
  Mux/1 -> Quaternions/1
  Product7/1 -> Add3/2
  Product6/1 -> Add3/1
  Product5/1 -> Add2/2
  Product4/1 -> Add2/1
  Product3/1 -> Add1/2
  Product2/1 -> Add1/1
  Product1/1 -> Add/2
  Product/1 -> Add/1
  Demux1/3 -> Product5/3, Product1/3, Product3/3, Product7/3  "cos(Y/2)"
  Demux1/1 -> Product5/1, Product2/1, Product1/1, Product6/1  "cos(R/2)"
  Demux1/2 -> Product6/2, Product1/2, Product3/2, Product4/2  "cos(P/2)"
  Trigonometric Function1/1 -> Demux1/1
  Demux/3 -> Product/3, Product2/3, Product4/3, Product6/3  "sin(Y/2)"
  Demux/2 -> Product/2, Product2/2, Product5/2, Product7/2  "sin(P/2)"
  Demux/1 -> Product/1, Product3/1, Product4/1, Product7/1  "sin(R/2)"
  Trigonometric Function/1 -> Demux/1
  Gain/1 -> Trigonometric Function/1, Trigonometric Function1/1
  "Euler Angles "/1 -> Gain/1

== system MJAUV_Maneuverability_model_V2/MJ-AUV Model & PropulsionSystem/Dynamics and Kinematics/Subsystem1 ==
  nu_B : Inport
  Theta : Inport  Port=2
  H_BS : Subsystem
  Matrix Multiply3 : Product  Multiplication=Matrix(*)
  Selector : Selector  InputPortWidth=3  IndexOptions=Index vector (dialog)  Indices=[1]  OutputSizes=1
  "{B}->{S} Transformation" : Subsystem
  nu_S : Outport
  wires:
  Matrix Multiply3/1 -> nu_S/1
  "{B}->{S} Transformation"/1(R(v)) -> H_BS/1(R_BS)  "R_BS"
  H_BS/1(H_BS) -> Matrix Multiply3/1
  Theta/1 -> Selector/1
  nu_B/1 -> Matrix Multiply3/2
  Selector/1 -> "{B}->{S} Transformation"/1(v)  "Theta1"

== system MJAUV_Maneuverability_model_V2/MJ-AUV Model & PropulsionSystem/Dynamics and Kinematics/Subsystem2 ==
  nu_S : Inport
  Theta : Inport  Port=2
  H_ST : Subsystem
  Matrix Multiply3 : Product  Multiplication=Matrix(*)
  Selector4 : Selector  InputPortWidth=3  IndexOptions=Index vector (dialog)  Indices=[2]  OutputSizes=1
  "{S}->{T} Transformation" : Subsystem
  nu_T : Outport
  wires:
  Matrix Multiply3/1 -> nu_T/1
  "{S}->{T} Transformation"/1(R(v)) -> H_ST/1(R_ST)  "R_ST"
  H_ST/1(H_ST) -> Matrix Multiply3/1
  Theta/1 -> Selector4/1
  nu_S/1 -> Matrix Multiply3/2
  Selector4/1 -> "{S}->{T} Transformation"/1(v)  "Theta2"

== system MJAUV_Maneuverability_model_V2/MJ-AUV Model & PropulsionSystem/Dynamics and Kinematics/Subsystem3 ==
  nu_T : Inport
  Theta : Inport  Port=2
  H_TF : Subsystem
  Matrix Multiply3 : Product  Multiplication=Matrix(*)
  Selector5 : Selector  InputPortWidth=3  IndexOptions=Index vector (dialog)  Indices=[3]  OutputSizes=1
  "{T}->{F} Transformation" : Subsystem
  nu_F : Outport
  wires:
  nu_T/1 -> Matrix Multiply3/2
  Theta/1 -> Selector5/1
  H_TF/1(H_TF) -> Matrix Multiply3/1
  "{T}->{F} Transformation"/1(R(v)) -> H_TF/1(R_TF)  "R_TF"
  Matrix Multiply3/1 -> nu_F/1
  Selector5/1 -> "{T}->{F} Transformation"/1(v)  "Theta3"

== system MJAUV_Maneuverability_model_V2/MJ-AUV Model & PropulsionSystem/Dynamics and Kinematics/Subsystem4 ==
  nu_B : Inport
  eta_E : Inport  Port=2
  Added Mass Coriolis and centripetal matrix : Subsystem
  Damping forces : Subsystem
  Matrix Multiply : Product  Multiplication=Matrix(*)
  Matrix Multiply2 : Product  Multiplication=Matrix(*)
  Restoring forces : Subsystem
  Rigid-body Coriolis and centripetal matrix : Subsystem
  g(eta_E)_B : Outport
  D_B * nu_B : Outport  Port=2
  CA_B * nu_B : Outport  Port=3
  CRB_B * nu_B : Outport  Port=4
  wires:
  nu_B/1 -> Added Mass Coriolis and centripetal matrix/1(nu_B), Matrix Multiply2/2, Damping forces/1(nu_B), Rigid-body Coriolis and centripetal matrix/1(nu_B), Matrix Multiply/2  "nu_B"
  Rigid-body Coriolis and centripetal matrix/1(CRB) -> Matrix Multiply/1
  Restoring forces/1(g(eta_E)_B) -> g(eta_E)_B/1
  eta_E/1 -> Restoring forces/1(eta_E)
  Matrix Multiply/1 -> CRB_B * nu_B/1
  Added Mass Coriolis and centripetal matrix/1(CA) -> Matrix Multiply2/1
  Damping forces/1(D * nu_B) -> D_B * nu_B/1
  Matrix Multiply2/1 -> CA_B * nu_B/1

== system MJAUV_Maneuverability_model_V2/MJ-AUV Model & PropulsionSystem/Dynamics and Kinematics/Subsystem5 ==
  Theta : Inport
  K : Subsystem
  K_B : Subsystem
  K_T : Subsystem
  Selector2 : Selector  InputPortWidth=3  IndexOptions=Index vector (dialog)  Indices=[1]  OutputSizes=1
  Selector3 : Selector  InputPortWidth=3  IndexOptions=Index vector (dialog)  Indices=[2]  OutputSizes=1
  Selector6 : Selector  InputPortWidth=3  IndexOptions=Index vector (dialog)  Indices=[3]  OutputSizes=1
  Transpose1 : matrix_library/Transpose
  Transpose2 : matrix_library/Transpose
  Transpose3 : matrix_library/Transpose
  "{B}->{S} Transformation" : Subsystem
  "{S}->{T} Transformation" : Subsystem
  "{T}->{F} Transformation" : Subsystem
  K_SB : Outport
  K_TS : Outport  Port=2
  K_FT : Outport  Port=3
  wires:
  Theta/1 -> Selector2/1, Selector3/1, Selector6/1
  K/1(K_FT) -> K_FT/1
  "{B}->{S} Transformation"/1(R(v)) -> Transpose3/1  "R_BS"
  Selector6/1 -> "{T}->{F} Transformation"/1(v)
  "{T}->{F} Transformation"/1(R(v)) -> Transpose1/1  "R_TF"
  Transpose3/1 -> K_B/1(R_SB)
  "{S}->{T} Transformation"/1(R(v)) -> Transpose2/1  "R_ST"
  Transpose2/1 -> K_T/1(R_TS)
  Selector2/1 -> "{B}->{S} Transformation"/1(v)
  Transpose1/1 -> K/1(R_FT)
  Selector3/1 -> "{S}->{T} Transformation"/1(v)
  K_B/1(K_SB) -> K_SB/1
  K_T/1(K_TS) -> K_TS/1

== system MJAUV_Maneuverability_model_V2/MJ-AUV Model & PropulsionSystem/Dynamics and Kinematics/Subsystem6 ==
  nu_S : Inport
  eta_E : Inport  Port=2
  Theta : Inport  Port=3
  In Bus Element2 : Inport  Port=4  PortName=uCMD  Element=rG_S
  Added Mass Coriolis and centripetal matrix1 : Subsystem
  Constant : Constant  Value=0
  Damping forces1 : Subsystem
  Matrix Multiply3 : Product  Multiplication=Matrix(*)
  Matrix Multiply4 : Product  Multiplication=Matrix(*)
  Restoring forces1 : Subsystem
      settings: PortSchema="{\"entries\":[{\"content\":{\"sides\":[{\"content\":{\"connectorIds\":[\"In1\"]},\"type\":\"ConnectorPlacement.EquallySpacedRectSide\",\"uuid\":\"0ea4a8db-38ae-4065-bd42-684e06b622e7\"},{\"content\":{\"connectorIds\":[\"Out1\"],\"side\":\"RIGHT\"},\"type\":\"ConnectorPlacement.EquallySpacedRectSide\",\"uuid\":\"a84d92ed-23bf-45f6-aee7-a752c5a7618c\"},{\"content\":{\"connectorIds\":[\"In2\"],\"side\":\"TOP\"},\"type\":\"ConnectorPlacement.EquallySpacedRectSide\",\"uuid\":\"7302fe7e-b448-4eb9-ba21-164e02ed0ef2\"}]},\"type\":\"ConnectorPlacement.EquallySpacedConnector\",\"uuid\":\"dd72758c-a98d-41ac-acc2-760c30b543d7\"}],\"packageUris\":[\"http://schema.mathworks.com/mf0/Connector/R2020b\"],\"version\":\"1.0\"}"
  Rigid-body Coriolis and centripetal matrix1 : Subsystem
      settings: PortSchema="{\"entries\":[{\"content\":{\"sides\":[{\"content\":{\"connectorIds\":[\"In1\"]},\"type\":\"ConnectorPlacement.EquallySpacedRectSide\",\"uuid\":\"36ccd2e0-0138-42d8-a792-30a059f1fcb3\"},{\"content\":{\"connectorIds\":[\"Out1\"],\"side\":\"RIGHT\"},\"type\":\"ConnectorPlacement.EquallySpacedRectSide\",\"uuid\":\"bc52fce8-ed6b-4915-ba7e-22ff9e979437\"},{\"content\":{\"connectorIds\":[\"In2\"],\"side\":\"TOP\"},\"type\":\"ConnectorPlacement.EquallySpacedRectSide\",\"uuid\":\"e9dd4bb6-e4cb-44b2-b6ba-42f5ec0171ee\"}]},\"type\":\"ConnectorPlacement.EquallySpacedConnector\",\"uuid\":\"2d6507b9-07e3-4b86-b480-134c98f22722\"}],\"packageUris\":[\"http://schema.mathworks.com/mf0/Connector/R2020b\"],\"version\":\"1.0\"}"
  Subsystem1 : Subsystem
  Sum2 : Sum  Inputs=|||+++++  SaturateOnIntegerOverflow=on
  (C+D)*nu + g : Outport
  wires:
  Matrix Multiply3/1 -> Sum2/3
  Damping forces1/1(D * nu_S) -> Sum2/4
  Added Mass Coriolis and centripetal matrix1/1(CA_S) -> Matrix Multiply3/1
  nu_S/1 -> Damping forces1/1(nu_S), Matrix Multiply3/2, Rigid-body Coriolis and centripetal matrix1/1(nu_S), Matrix Multiply4/2, Added Mass Coriolis and centripetal matrix1/1(nu_S)
  Rigid-body Coriolis and centripetal matrix1/1(CRB_S) -> Matrix Multiply4/1
  Restoring forces1/1(g(eta_E)_S) -> Sum2/5
  Matrix Multiply4/1 -> Sum2/2
  Sum2/1 -> (C+D)*nu + g/1  "(C+D)*nu + g"
  Constant/1 -> Sum2/1
  eta_E/1 -> Subsystem1/1(eta_E_B)
  Theta/1 -> Subsystem1/2(Theta)
  Subsystem1/1(eta_E_S) -> Restoring forces1/1(eta_E)
  In Bus Element2/1 -> Restoring forces1/2(rG_S), Rigid-body Coriolis and centripetal matrix1/2(rG_S)

== system MJAUV_Maneuverability_model_V2/MJ-AUV Model & PropulsionSystem/Dynamics and Kinematics/Subsystem7 ==
  nu_T : Inport
  eta_E : Inport  Port=2
  Theta : Inport  Port=3
  In Bus Element2 : Inport  Port=4  PortName=uCMD  Element=Delta_B_T
  Added Mass Coriolis and centripetal matrix1 : Subsystem
  B_T0 : Constant  Value=498.45
  Constant : Constant  Value=0
  Damping forces1 : Subsystem
  Matrix Multiply3 : Product  Multiplication=Matrix(*)
  Matrix Multiply4 : Product  Multiplication=Matrix(*)
  Restoring forces1 : Subsystem
      settings: PortSchema="{\"entries\":[{\"content\":{\"sides\":[{\"content\":{\"connectorIds\":[\"In1\"]},\"type\":\"ConnectorPlacement.EquallySpacedRectSide\",\"uuid\":\"36ccd2e0-0138-42d8-a792-30a059f1fcb3\"},{\"content\":{\"connectorIds\":[\"Out1\"],\"side\":\"RIGHT\"},\"type\":\"ConnectorPlacement.EquallySpacedRectSide\",\"uuid\":\"bc52fce8-ed6b-4915-ba7e-22ff9e979437\"},{\"content\":{\"connectorIds\":[],\"side\":\"TOP\"},\"type\":\"ConnectorPlacement.EquallySpacedRectSide\",\"uuid\":\"e9dd4bb6-e4cb-44b2-b6ba-42f5ec0171ee\"},{\"content\":{\"connectorIds\":[\"In2\"],\"side\":\"BOTTOM\"},\"type\":\"ConnectorPlacement.EquallySpacedRectSide\",\"uuid\":\"a738e7a3-55f8-4cb2-894a-eb8b6d84b0d6\"}]},\"type\":\"ConnectorPlacement.EquallySpacedConnector\",\"uuid\":\"2d6507b9-07e3-4b86-b480-134c98f22722\"}],\"packageUris\":[\"http://schema.mathworks.com/mf0/Connector/R2020b\"],\"version\":\"1.0\"}"
  Rigid-body Coriolis and centripetal matrix1 : Subsystem
  Subsystem1 : Subsystem
  Sum : Sum  Inputs=|++
  Sum2 : Sum  Inputs=||||+++++  SaturateOnIntegerOverflow=on
  (C+D)*nu + g : Outport
  wires:
  Subsystem1/1(eta_E_T) -> Restoring forces1/1(eta_E)
  Matrix Multiply4/1 -> Sum2/2
  Restoring forces1/1(g(eta_E)_T) -> Sum2/5
  Rigid-body Coriolis and centripetal matrix1/1(CRB_T) -> Matrix Multiply4/1
  Added Mass Coriolis and centripetal matrix1/1(CA_T) -> Matrix Multiply3/1
  Damping forces1/1(D * nu_T) -> Sum2/4
  Matrix Multiply3/1 -> Sum2/3
  Sum2/1 -> (C+D)*nu + g/1  "(C+D)*nu + g"
  nu_T/1 -> Added Mass Coriolis and centripetal matrix1/1(nu_T), Matrix Multiply4/2, Rigid-body Coriolis and centripetal matrix1/1(nu_T), Matrix Multiply3/2, Damping forces1/1(nu_T)
  Constant/1 -> Sum2/1
  Theta/1 -> Subsystem1/2(Theta)
  eta_E/1 -> Subsystem1/1(eta_E_B)
  In Bus Element2/1 -> Sum/1
  B_T0/1 -> Sum/2
  Sum/1 -> Restoring forces1/2(B_T)  "B_T"

== system MJAUV_Maneuverability_model_V2/MJ-AUV Model & PropulsionSystem/Dynamics and Kinematics/Subsystem8 ==
  nu_F : Inport
  eta_E : Inport  Port=2
  Theta : Inport  Port=3
  Added Mass Coriolis and centripetal matrix1 : Subsystem
  Constant : Constant  Value=0
  Damping forces1 : Subsystem
  Matrix Multiply3 : Product  Multiplication=Matrix(*)
  Matrix Multiply4 : Product  Multiplication=Matrix(*)
  Restoring forces1 : Subsystem
  Rigid-body Coriolis and centripetal matrix1 : Subsystem
  Subsystem1 : Subsystem
  Sum2 : Sum  Inputs=|||+++++  SaturateOnIntegerOverflow=on
  (C+D)*nu + g : Outport
  wires:
  Matrix Multiply3/1 -> Sum2/3
  Damping forces1/1(D * nu_F) -> Sum2/4
  Added Mass Coriolis and centripetal matrix1/1(CA_F) -> Matrix Multiply3/1
  Rigid-body Coriolis and centripetal matrix1/1(CRB_F) -> Matrix Multiply4/1
  Restoring forces1/1(g(eta_E)_T) -> Sum2/5
  Matrix Multiply4/1 -> Sum2/2
  Sum2/1 -> (C+D)*nu + g/1  "(C+D)*nu + g"
  nu_F/1 -> Damping forces1/1(nu_F), Matrix Multiply3/2, Rigid-body Coriolis and centripetal matrix1/1(nu_F), Matrix Multiply4/2, Added Mass Coriolis and centripetal matrix1/1(nu_F)
  Constant/1 -> Sum2/1
  Theta/1 -> Subsystem1/2(Theta)
  eta_E/1 -> Subsystem1/1(eta_E_B)
  Subsystem1/1(eta_E_T) -> Restoring forces1/1(eta_E)

== system MJAUV_Maneuverability_model_V2/MJ-AUV Model & PropulsionSystem/Dynamics and Kinematics/Subsystem9 ==
  In1 : Inport
  In Bus Element1 : Inport  Port=2  PortName=uCMD  Element=Theta
  In Bus Element2 : Inport  Port=2  PortName=uCMD  Element=rG_S
  Divide : Product  Inputs=*/  Multiplication=Matrix(*)
  M_B : Subsystem
  M_F : Subsystem
  M_S : Subsystem
      settings: PortSchema="{\"entries\":[{\"content\":{\"sides\":[{\"content\":{\"connectorIds\":[]},\"type\":\"ConnectorPlacement.EquallySpacedRectSide\",\"uuid\":\"882279a2-f725-41a9-aa2b-b51267a1cbf1\"},{\"content\":{\"connectorIds\":[\"Out1\"],\"side\":\"RIGHT\"},\"type\":\"ConnectorPlacement.EquallySpacedRectSide\",\"uuid\":\"723bed1e-b1cb-4096-89b3-c9ba2b7a3134\"},{\"content\":{\"connectorIds\":[],\"side\":\"TOP\"},\"type\":\"ConnectorPlacement.EquallySpacedRectSide\",\"uuid\":\"9485ee79-5489-45d8-94d5-ac1750625f3a\"},{\"content\":{\"connectorIds\":[\"In1\"],\"side\":\"BOTTOM\"},\"type\":\"ConnectorPlacement.EquallySpacedRectSide\",\"uuid\":\"2e4d3e44-6553-4d5f-b245-ae1a573616b1\"}]},\"type\":\"ConnectorPlacement.EquallySpacedConnector\",\"uuid\":\"ffc7b5c8-b897-4313-becf-8eac0d6fa409\"}],\"packageUris\":[\"http://schema.mathworks.com/mf0/Connector/R2020b\"],\"version\":\"1.0\"}"
  M_T : Subsystem
  Matrix Multiply{1,3..5} (4 alike) : Product  Multiplication=Matrix(*)
  Matrix Multiply2 : Product  Inputs=3  Multiplication=Matrix(*)
  Subsystem5 : Subsystem
  Sum : Sum  Inputs=|++++
  Transpose : matrix_library/Transpose
  nudot : Outport
  wires:
  Divide/1 -> nudot/1  "nudot"
  Matrix Multiply2/1 -> Matrix Multiply5/1
  Matrix Multiply1/1 -> Matrix Multiply4/1, Matrix Multiply2/2
  M_S/1(M_S) -> Matrix Multiply3/2
  M_T/1(M_T) -> Matrix Multiply4/2
  M_F/1(M_F) -> Matrix Multiply5/2
  M_B/1(M_B) -> Sum/1
  Matrix Multiply3/1 -> Sum/2
  Matrix Multiply4/1 -> Sum/3
  Matrix Multiply5/1 -> Sum/4
  In1/1 -> Transpose/1
  Sum/1 -> Divide/2
  Transpose/1 -> Divide/1
  In Bus Element1/1 -> Subsystem5/1(Theta)
  Subsystem5/3(K_SB) -> Matrix Multiply1/2, Matrix Multiply2/3, Matrix Multiply3/1
  Subsystem5/2(K_TS) -> Matrix Multiply1/1  "K_TS"
  Subsystem5/1(K_FT) -> Matrix Multiply2/1  "K_FT"
  In Bus Element2/1 -> M_S/1(rG_S)

== system MJAUV_Maneuverability_model_V2/MJ-AUV Model & PropulsionSystem/Propulsion System/Horizontal Force and Moment (Tau_H) ==
  note: U=modulo(u v w)
  uHT : Inport
  nu_B : Inport  Port=2
  Abs : Abs  SaturateOnIntegerOverflow=off
  Abs1 : Abs  SaturateOnIntegerOverflow=off
  Dot Product : DotProduct  OutDataTypeStr=Inherit: Inherit via internal rule
  Gain1 : Gain  Gain=0.4421
  Gain3 : Gain  Gain=D
  HT_prop : Constant  Value=K_prop
  KT_VT1 : Fcn  Expr=-0.4674*u(1)*u(2)
  KT_VT2 : Fcn  Expr=0.4674*u(1)*u(2)
  Matrix Multiply : Product  Multiplication=Matrix(*)
  Mux3 : Mux  Inputs=2
  Product : Product
  Selector : Selector  InputPortWidth=6  IndexOptions=Index vector (dialog)  Indices=[1 2 3]  OutputSizes=1
  Sqrt : Sqrt
  Sum2 : Sum  Inputs=|++
  Switch : Switch  Criteria=u2 > Threshold  SaturateOnIntegerOverflow=off  InputSameDT=off
  Tau_HT : Outport
  wires:
  Product/1 -> Gain1/1
  Mux3/1 -> KT_VT1/1, KT_VT2/1
  Gain1/1 -> Gain3/1
  HT_prop/1 -> Matrix Multiply/1
  Dot Product/1 -> Sqrt/1
  Sqrt/1 -> Mux3/2
  Sum2/1 -> Matrix Multiply/2
  Matrix Multiply/1 -> Tau_HT/1  "[surge_HT1 0 0 0 0 0]"
  Selector/1 -> Dot Product/1, Dot Product/2
  uHT/1 -> Abs/1, Product/2, Abs1/1, Switch/2
  Abs1/1 -> Product/1
  KT_VT1/1 -> Switch/1
  nu_B/1 -> Selector/1
  Switch/1 -> Sum2/2
  Gain3/1 -> Sum2/1
  Abs/1 -> Mux3/1
  KT_VT2/1 -> Switch/3

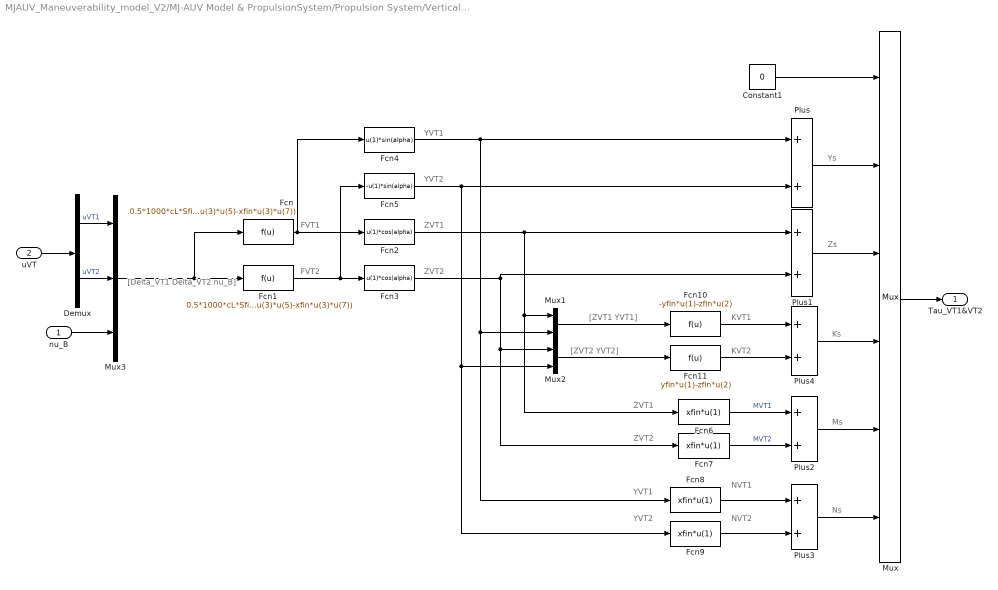
== system MJAUV_Maneuverability_model_V2/MJ-AUV Model & PropulsionSystem/Propulsion System/Vertical Force and Moment (Tau_V) ==
  note: Ks
  note: YVT2
  note: Zs
  note: YVT1
  note: [ZVT2 YVT2]
  note: ZVT1
  note: ZVT1
  note: ZVT2
  note: NVT2
  note: KVT2
  note: KVT1
  note: NVT1
  note: FVT2
  note: YVT2
  note: Ms
  note: [Delta_VT1 Delta_VT2 nu_B]
  note: FVT1
  note: [ZVT1 YVT1]
  note: Ns
  note: YVT1
  note: ZVT2
  note: Ys
  nu_B : Inport
  uVT : Inport  Port=2
  Constant1 : Constant  Value=0
  Demux : Demux  Outputs=2
  Fcn : Fcn  Expr=0.5*1000*cL*Sfin*(u(3)^2*u(1)+u(3)*u(5)-xfin*u(3)*u(7))
  Fcn1 : Fcn  Expr=0.5*1000*cL*Sfin*(u(3)^2*u(2)+u(3)*u(5)-xfin*u(3)*u(7))
  Fcn10 : Fcn  Expr=-yfin*u(1)-zfin*u(2)
  Fcn11 : Fcn  Expr=yfin*u(1)-zfin*u(2)
  Fcn2 : Fcn  Expr=u(1)*cos(alpha)
  Fcn3 : Fcn  Expr=u(1)*cos(alpha)
  Fcn4 : Fcn  Expr=u(1)*sin(alpha)
  Fcn5 : Fcn  Expr=-u(1)*sin(alpha)
  Fcn{6..9} (4 alike) : Fcn  Expr=xfin*u(1)
  Mux : Mux  Inputs=6
  Mux1 : Mux  Inputs=2
  Mux2 : Mux  Inputs=2
  Mux3 : Mux  Inputs=3
  Plus{,1..4} (5 alike) : Sum
  "Tau_VT1&VT2 " : Outport  VectorParamsAs1DForOutWhenUnconnected=off
  wires:
  Fcn2/1 -> Plus1/1, Fcn6/1, Mux1/1
  Mux/1 -> "Tau_VT1&VT2 "/1
  Fcn1/1 -> Fcn3/1, Fcn5/1
  Fcn/1 -> Fcn2/1, Fcn4/1
  Fcn5/1 -> Plus/2, Fcn9/1, Mux2/2
  Fcn9/1 -> Plus3/2
  Plus4/1 -> Mux/4
  Mux2/1 -> Fcn11/1
  Fcn3/1 -> Fcn7/1, Mux2/1, Plus1/2
  Constant1/1 -> Mux/1
  Plus/1 -> Mux/2
  Mux1/1 -> Fcn10/1
  Plus2/1 -> Mux/5
  Fcn10/1 -> Plus4/1
  Fcn4/1 -> Fcn8/1, Mux1/2, Plus/1
  nu_B/1 -> Mux3/3
  Plus1/1 -> Mux/3
  Fcn11/1 -> Plus4/2
  Fcn8/1 -> Plus3/1
  Plus3/1 -> Mux/6
  Mux3/1 -> Fcn1/1, Fcn/1
  Fcn6/1 -> Plus2/1  "MVT1"
  Fcn7/1 -> Plus2/2  "MVT2"
  Demux/2 -> Mux3/2  "uVT2"
  Demux/1 -> Mux3/1  "uVT1"
  uVT/1 -> Demux/1
